simulink model "35 Bus Network Electricity Transmission Model"  (R2023b)
settings: Solver=VariableStepAuto  StartTime=0.0  StopTime=1  RelTol=1e-3
model workspace (MAT data in the model file):
  T_set = 0.0001
  Tp = 5e-05
undefined symbols (not defined in the file): D1, D11, Delta, DiscIntNeverNeededParam
libraries: spsSeriesRLCBranchLib x57, spsLoadFlowBusLib x35, spsThreePhaseSeriesRLCLoadLib x28, spsThreePhaseTransformerTwoWindingsLib x22, spsDistributedParametersLineLib x22, spsGenericPowerSystemStabilizerLib x20, spsThreePhaseVIMeasurementLib x14, spsSynchronousMachinepuStandardLib x10, spsExcitationSystemLib x10, spsHydraulicTurbineandGovernorLib x10, spsFourierLib x8, spsMeanLib x8
(part 4 of 8)

== system 35 Bus Network Electricity Transmission Model/Regulators 10 ==
  m : Inport
  Bus Selector : BusSelector  OutputSignals="dq0 components.Stator voltage  vq (pu),dq0 components.Stator voltage  vd (pu),Mechanical.Rotor speed  wm  (pu),Output active power   Peo (pu)"
  Constant : Constant  Value=0.81818
  Constant1 : Constant
  Math Function : Math  Operator=hypot
  Turbine and Excitation Regulators : Subsystem
  Pm : Outport
  Vf : Outport  Port=2
  tag scope: Vm10=global, w10=global
  wires:
  Bus Selector/4 -> Turbine and Excitation Regulators/3(Pe 0)  "<Output active power   Peo (pu)>"
  Constant1/1 -> Turbine and Excitation Regulators/4(Vref)
  Bus Selector/3 -> [w10], Turbine and Excitation Regulators/2(w)  "<Rotor speed  wm  (pu)>"
  Turbine and Excitation Regulators/1(Pm) -> Pm/1
  m/1 -> Bus Selector/1
  Turbine and Excitation Regulators/2(Vf) -> Vf/1
  Bus Selector/2 -> Math Function/1  "<Stator voltage  vd (pu)>"
  Math Function/1 -> [Vm10], Turbine and Excitation Regulators/5(Vm)
  Bus Selector/1 -> Math Function/2  "<Stator voltage  vq (pu)>"
  Constant/1 -> Turbine and Excitation Regulators/1(pref)
